simulink model "Main_Project"  (R2016a)
settings: Solver=ode4  StartTime=0.0  StopTime=100  FixedStep=0.001  MaxStep=0.01  RelTol=1e-6
values from neighbouring files (symbols this model uses):
  float =     [waveglider.mat]
  floatABC =     [waveglider.mat]
  gliderABC =     [waveglider.mat]
undefined symbols (not defined in the file or in its folder): magnitude, RAO_Vel
libraries: simulink_extras x8, marine_gnc x4, simulink x4, marine_hydro x1
(part 2 of 3)

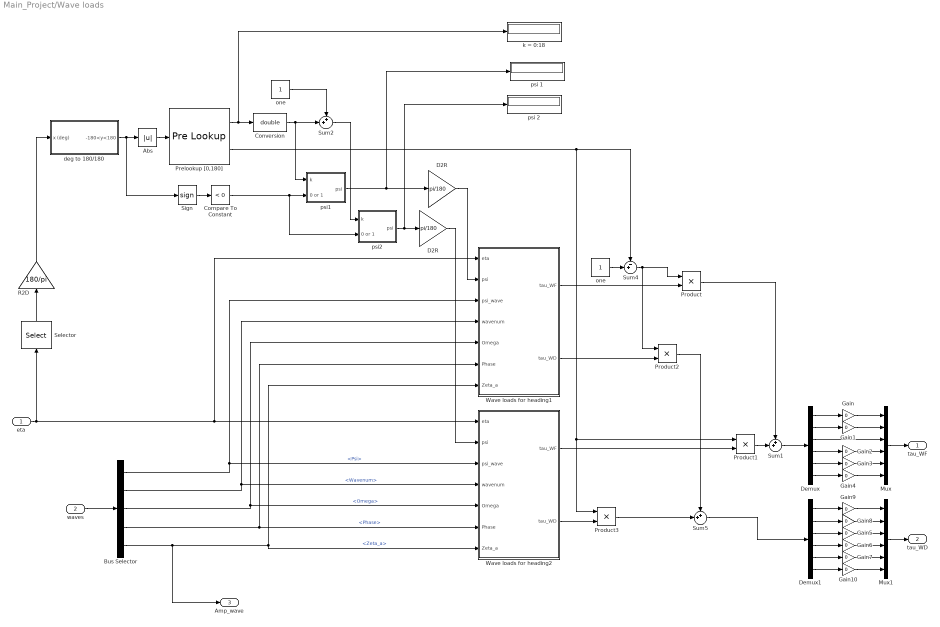
== system Main_Project/Wave loads ==
  eta : Inport
  waves : Inport  Port=2
  Abs : Abs  SaturateOnIntegerOverflow=on
  Bus Selector : BusSelector  OutputSignals=Psi,Wavenum,Omega,Phase,Zeta_a
  Compare To Constant : simulink/Logic and Bit Operations/Compare To Constant  relop=<  const=0  OutDataTypeStr=uint8  ZeroCross=off
  Conversion : DataTypeConversion  OutDataTypeStr=double
  D2R : Gain  Gain=pi/180
  "D2R " : Gain  Gain=pi/180
  Demux : Demux  Outputs=6
  Demux1 : Demux  Outputs=6
  Gain{,1..10} (11 alike) : Gain  Gain=0
  Mux : Mux  Inputs=6
  Mux1 : Mux  Inputs=6
  Prelookup [0,180] : PreLookup  BreakpointsData=[0:10:180]  IndexSearchMethod=Evenly spaced points  BeginIndexSearchUsingPreviousIndexResult=on
  Product{,1..3} (4 alike) : Product  RndMeth=Zero
  R2D : Gain  Gain=180/pi
  Selector : Selector  InputPortWidth=6  IndexOptions=Index vector (dialog)  Indices=[6]  OutputSizes=1
  Sign : Signum
  Sum1 : Sum  Inputs=++|
  Sum2 : Sum  Inputs=++|
  Sum4 : Sum  Inputs=-+|
  Sum5 : Sum  Inputs=++|
  Wave loads for heading1 : Subsystem  mask(Force RAO){ForceRAO_Freq=float.forceRAO.w, WD_Freq=float.driftfrc.w, ForceRAO_Amp=float.forceRAO.amp, ForceRAO_Phase=float.forceRAO.phase, WD_Amp=float.driftfrc.amp, RAO_add_omega_0=on, RAO_add_omega_inf=on}
      mask prompts: ForceRAO_Freq "Vector of frequencies ForceRAO_Freq (rad/s)"; WD_Freq "Vector of frequencies WD_Freq (rad/s)"; ForceRAO_Amp "6DOF Cell array with tables of Amplitudes ForceRAO_Amp"; ForceRAO_Phase "6DOF Cell array with tables of Phases ForceRAO_Phase (rad)"; WD_Amp "6DOF Cell array with tables of Amplitudes WD_Amp"; RAO_add_omega_0 "Add asymptotic RAO values for omega = 0"; RAO_add_omega_inf "Add asymptotic RAO values for omega = inf"
      mask help:
      | Calculate the 6 degrees-of-freedom (DOF) wave-frequency excitation forces tau_WF for a vessel from its Force Response Amplitude Operators (Force RAOs) and a sea state defined by a set of harmonic waves. The block takes the "Waves" bus from the MSS Waves block as input, as well as the vessel low-frequency (LF) motion in terms of the generalized position vector eta and mean surge velocity U. See help for details.
      |
      | Authors: Oyvind N. Smogeli and Thor I. Fossen, 2005-05-03
      mask Help:
      | <b>Part of the Marine Systems Simulator: MSS</b><br>
      | <br>
      | Calculate the 6 degrees-of-freedom (DOF) wave-frequency excitation forces tau_WF
      | for a vessel from its Force Response Amplitude Operators (Force RAOs) and a sea
      | state defined by a set of harmonic waves. The block takes the &quot;Waves&quot; bus from
      | the MSS Waves block as input, as well as the vessel low-frequency (LF) motion in
      | terms of the generalized position vector eta and mean surge velocity U.<p>The Force RAOs are defined in terms of a
      | vector of frequencies (RAO_Freq), a vector of directions (RAO_Dir), a vector of
      | velocities (RAO_Dir), a 6DOF cell array of 3D matrices with amplitudes
      | (RAO_Amp), and a 6DOF cell array of 3D matrices with phases (RAO_Phase), which
      | are all input in the block mask. The first dimension of the 3D matrices
      | corresponds to the frequencies, the second to the directions, and the third to
      | the velocities, such that e.g. the amplitude amp in heave (DOF #3) for frequency
      | number n_f, direction number n_d and velocity number n_v can be found from a =
      | RAO_Amp{3}(n_f, n_d, n_v).</p>
      | <p><b>Inputs:</b></p>
      | <p>Waves:&nbsp;&nbsp;&nbsp;&nbsp;&nbsp;&nbsp;&nbsp;&nbsp;&nbsp;&nbsp;&nbsp; Bus
      | containing the following signals<br>
      | &nbsp;&nbsp;&nbsp; Zeta_a:&nbsp;&nbsp;&nbsp;&nbsp;&nbsp;&nbsp;&nbsp; Vector of harmonic wave amplitudes [m]<br>
      | &nbsp;&nbsp;&nbsp; Omega:&nbsp;&nbsp;&nbsp;&nbsp;&nbsp;&nbsp; Vector of harmonic wave frequencies [rad/s]<br>
      | &nbsp;&nbsp;&nbsp; Phase:&nbsp;&nbsp;&nbsp;&nbsp;&nbsp;&nbsp;&nbsp;&nbsp; Vector of harmonic wave phases (random) [rad]<br>
      | &nbsp;&nbsp;&nbsp; Wavenum:&nbsp;&nbsp;&nbsp; Vector of harmonic wave numbers [1/m]<br>
      | &nbsp;&nbsp;&nbsp; Psi:&nbsp;&nbsp;&nbsp;&nbsp;&nbsp;&nbsp;&nbsp;&nbsp;&nbsp;&nbsp;&nbsp;&nbsp;&nbsp; Vector of harmonic wave directions [rad]</p>
      | <p>eta_LF:&nbsp;&nbsp;&nbsp;&nbsp;&nbsp;&nbsp;&nbsp;&nbsp;&nbsp;&nbsp;&nbsp;
      | Generalized 6DOF n-frame low-frequency position vector [x (m), y (m), z (m),
      | theta (rad), phi (rad), psi (rad)]<br>
      | U:&nbsp;&nbsp;&nbsp;&nbsp;&nbsp;&nbsp;&nbsp;&nbsp;&nbsp;&nbsp;&nbsp;&nbsp;&nbsp;&nbsp;&nbsp;&nbsp;&nbsp;&nbsp;&nbsp;
      | Low-frequency (mean) surge velocity&nbsp; [m/s]</p>
      | <p><b>Outputs:</b></p>
      | <p>tau_WF:&nbsp;&nbsp;&nbsp;&nbsp;&nbsp;&nbsp;&nbsp;&nbsp;&nbsp; Generalized
      | 6DOF h-frame force vector [X (N), Y (N), Z (N), K (Nm), M (Nm), N (Nm)]</p>
      | <p><b>Model validity:</b></p>
      | <p>The validity of the block is dependent on the validity of the given
      | RAO data set.</p>
      | <p>A proper RAO to be used with this block should contain at least 1 velocity, 5
      | directions (e.g. 0, 45, 90, 135 and 180 degrees) and 10-20 frequencies, for all
      | 6 DOF (surge, sway, heave, roll, pitch, yaw).</p>
      | <p>The block performs linear interpolation in frequencies and directions, and
      | uses the data set for the velocity closest to the input velocity (i.e. 'nearest'
      | interpolation in velocity). If the block recieves an input wave frequency or relative
      | wave direction outside the span of the data vectors RAO_Freq or RAO_Dir
      | respectively, the simulation stops and an error is returned. This means that a well-defined
      | RAO must contain data for both 0 and 180 degrees, and for frequencies covering
      | the desired range of wave frequencies. If desired, asymptotic values can be
      | automatically added for zero and infinity frequency to avoid runtime errors if
      | the wave freqeuncy exceeds the values in RAO_Freq (see checkboxes in the mask). </p>
      | <p>IMPORTANT NOTE: The RAO theory upon which this block is based is in reality
      | only valid when the vessel low-frequency (h-frame) motion is a constant surge
      | velocity only, and the vessel is performing wave-frequency oscillations about
      | the steadily translating h-frame.This means that the outputs from the block when
      | manoeuvering -- i.e. changing the surge velocity and/or yaw angle -- must be
      | interpreted with some care. A jump in the output must be expected when changing
      | between two velocity data sets, and frequency warping expected when changing the
      | yaw angle (due to interpolation in the phase). It is therefore recommended to
      | use backlash on the input velocity to avoid transient switching, and a quantized
      | yaw angle with backlash. The latter will lead to jump in the ouput when the yaw
      | angle changes from one quantized value to another, but will give better results
      | when keeping within one quantizer interval. The quantized yaw angle with
      | backlash and velocity with backlash are available as options via checkboxes in
      | the mask. If either of these are activated, proper values for the yaw
      | quantization interval, yaw backlash width, and the the speed backlash width
      | respectively must be set. Typical values could be a yaw quantization interval of
      | 5 degrees, yaw backlash width of 1/4-1/5 of the quantization interval, and speed
      | backlash width of 1 m/s. To avoid the most rapid transients when switching
      | between data sets, output smoothing is available as an option in the mask. If
      | this is enabled, the output during a transent is rate limited according to the
      | fastest recorded signal rate during normal operation.</p>
      | <p><b>Example mask input:</b></p><p>
      | As an example, the format of the mask input for 2 velocities, 3 directions and 5
      | frequencies is as follows:<p>RAO_Freq = [f1 f2 f3 f4 f5]<br>
      | RAO_Dir = [d1 d2 d3]<br>
      | RAO_Vel = [v1 v2]<p>Surge:<br>
      | RAO_Amp{1}(:,:,1)&nbsp; = [a1_111 a1_121 a1_131; a1_211 a1_221 a1_231; a1_311
      | a1_321 a1_331; a1_411 a1_421 a1_431; a1_511 a1_521 a1_531]<br>
      | RAO_Amp{1}(:,:,2)&nbsp; = [a1_112 a1_122 a1_132; a1_212 a1_222 a1_232; a1_312
      | a1_322 a1_332; a1_412 a1_422 a1_432; a1_512 a1_522 a1_532]<br>
      | RAO_Phase{1}(:,:,1) = [p1_111 p1_121 p1_131; p1_211 p1_221 p1_231; p1_311 p1_321
      | p1_331; p1_411 p1_421 p1_431; p1_511 p1_521 p1_531]<br>
      | RAO_Phase{1}(:,:,2) = [p1_112 p1_122 p1_132; p1_212 p1_222 p1_232; p1_312 p1_322
      | p1_332; p1_412 p1_422 p1_432; p1_512 p1_522 p1_532]<p>Sway:<br>
      | RAO_Amp{2}(:,:,1)&nbsp; = [a2_111 a2_121 a2_131; a2_211 a2_221 a2_231; a2_311
      | a2_321 a2_331; a2_411 a2_421 a2_431; a2_511 a2_521 a2_531]<br>
      | RAO_Amp{2}(:,:,2)&nbsp; = [a2_112 a2_122 a2_132; a2_212 a2_222 a2_232; a2_312
      | a2_322 a2_332; a2_412 a2_422 a2_432; a2_512 a2_522 a2_532]<br>
      | RAO_Phase{2}(:,:,1) = [p2_111 p2_121 p2_131; p2_211 p2_221 p2_231; p2_311 p2_321
      | p2_331; p2_411 p2_421 p2_431; p2_511 p2_521 p2_531]<br>
      | RAO_Phase{2}(:,:,2) = [p2_112 p2_122 p2_132; p2_212 p2_222 p2_232; p2_312 p2_322
      | p2_332; p2_412 p2_422 p2_432; p2_512 p2_522 p2_532]<p>...<p>Yaw:<br>
      | RAO_Amp{6}(:,:,1)&nbsp; = [a6_111 a6_121 a6_131; a6_211 a6_221 a6_231; a6_311
      | a6_321 a6_331; a6_411 a6_421 a6_431; a6_511 a6_521 a6_531]<br>
      | RAO_Amp{6}(:,:,2)&nbsp; = [a6_112 a6_122 a6_132; a6_212 a6_222 a6_232; a6_312
      | a6_322 a6_332; a6_412 a6_422 a6_432; a6_512 a6_522 a6_532]<br>
      | RAO_Phase{6}(:,:,1) = [p6_111 p6_121 p6_131; p6_211 p6_221 p6_231; p6_311 p6_321
      | p6_331; p6_411 p6_421 p6_431; p6_511 p6_521 p6_531]<br>
      | RAO_Phase{6}(:,:,2) = [p6_112 p6_122 p6_132; p6_212 p6_222 p6_232; p6_312 p6_322
      | p6_332; p6_412 p6_422 p6_432; p6_512 p6_522 p6_532]<p>where now for example the
      | amplitude and phase in sway (DOF 2) for frequency f5, direction d3 and velocity
      | v1 are given by RAO_Amp{2}(5,3,1) = a2_531 and RAO_Phase{2}(5,3,1) = p2_531.<p>
      | <b>Copyright (C) NTNU 2005</b></p>
      | <p><b>Author:</b> Oyvind N. Smogeli, 2005-05-03</p>
  Wave loads for heading2 : Subsystem  mask(Force RAO){ForceRAO_Freq=float.forceRAO.w, RAO_Vel=float.velocities, ForceRAO_Amp=float.forceRAO.amp, ForceRAO_Phase=float.forceRAO.phase, WD_Amp=float.driftfrc.amp, RAO_add_omega_0=on, RAO_add_omega_inf=on}
      mask prompts: ForceRAO_Freq "Vector of frequencies ForceRAO_Freq (rad/s)"; RAO_Vel "Vector of velocities RAO_Vel (m/s)"; ForceRAO_Amp "6DOF Cell array with tables of Amplitudes ForceRAO_Amp"; ForceRAO_Phase "6DOF Cell array with tables of Phases ForceRAO_Phase (rad)"; WD_Amp "6DOF Cell array with tables of Amplitudes WD_Amp"; RAO_add_omega_0 "Add asymptotic RAO values for omega = 0"; RAO_add_omega_inf "Add asymptotic RAO values for omega = inf"
      mask help:
      | Calculate the 6 degrees-of-freedom (DOF) wave-frequency excitation forces tau_WF for a vessel from its Force Response Amplitude Operators (Force RAOs) and a sea state defined by a set of harmonic waves. The block takes the "Waves" bus from the MSS Waves block as input, as well as the vessel low-frequency (LF) motion in terms of the generalized position vector eta and mean surge velocity U. See help for details.
      |
      | Authors: Oyvind N. Smogeli and Thor I. Fossen, 2005-05-03
      mask Help:
      | <b>Part of the Marine Systems Simulator: MSS</b><br>
      | <br>
      | Calculate the 6 degrees-of-freedom (DOF) wave-frequency excitation forces tau_WF
      | for a vessel from its Force Response Amplitude Operators (Force RAOs) and a sea
      | state defined by a set of harmonic waves. The block takes the &quot;Waves&quot; bus from
      | the MSS Waves block as input, as well as the vessel low-frequency (LF) motion in
      | terms of the generalized position vector eta and mean surge velocity U.<p>The Force RAOs are defined in terms of a
      | vector of frequencies (RAO_Freq), a vector of directions (RAO_Dir), a vector of
      | velocities (RAO_Dir), a 6DOF cell array of 3D matrices with amplitudes
      | (RAO_Amp), and a 6DOF cell array of 3D matrices with phases (RAO_Phase), which
      | are all input in the block mask. The first dimension of the 3D matrices
      | corresponds to the frequencies, the second to the directions, and the third to
      | the velocities, such that e.g. the amplitude amp in heave (DOF #3) for frequency
      | number n_f, direction number n_d and velocity number n_v can be found from a =
      | RAO_Amp{3}(n_f, n_d, n_v).</p>
      | <p><b>Inputs:</b></p>
      | <p>Waves:&nbsp;&nbsp;&nbsp;&nbsp;&nbsp;&nbsp;&nbsp;&nbsp;&nbsp;&nbsp;&nbsp; Bus
      | containing the following signals<br>
      | &nbsp;&nbsp;&nbsp; Zeta_a:&nbsp;&nbsp;&nbsp;&nbsp;&nbsp;&nbsp;&nbsp; Vector of harmonic wave amplitudes [m]<br>
      | &nbsp;&nbsp;&nbsp; Omega:&nbsp;&nbsp;&nbsp;&nbsp;&nbsp;&nbsp; Vector of harmonic wave frequencies [rad/s]<br>
      | &nbsp;&nbsp;&nbsp; Phase:&nbsp;&nbsp;&nbsp;&nbsp;&nbsp;&nbsp;&nbsp;&nbsp; Vector of harmonic wave phases (random) [rad]<br>
      | &nbsp;&nbsp;&nbsp; Wavenum:&nbsp;&nbsp;&nbsp; Vector of harmonic wave numbers [1/m]<br>
      | &nbsp;&nbsp;&nbsp; Psi:&nbsp;&nbsp;&nbsp;&nbsp;&nbsp;&nbsp;&nbsp;&nbsp;&nbsp;&nbsp;&nbsp;&nbsp;&nbsp; Vector of harmonic wave directions [rad]</p>
      | <p>eta_LF:&nbsp;&nbsp;&nbsp;&nbsp;&nbsp;&nbsp;&nbsp;&nbsp;&nbsp;&nbsp;&nbsp;
      | Generalized 6DOF n-frame low-frequency position vector [x (m), y (m), z (m),
      | theta (rad), phi (rad), psi (rad)]<br>
      | U:&nbsp;&nbsp;&nbsp;&nbsp;&nbsp;&nbsp;&nbsp;&nbsp;&nbsp;&nbsp;&nbsp;&nbsp;&nbsp;&nbsp;&nbsp;&nbsp;&nbsp;&nbsp;&nbsp;
      | Low-frequency (mean) surge velocity&nbsp; [m/s]</p>
      | <p><b>Outputs:</b></p>
      | <p>tau_WF:&nbsp;&nbsp;&nbsp;&nbsp;&nbsp;&nbsp;&nbsp;&nbsp;&nbsp; Generalized
      | 6DOF h-frame force vector [X (N), Y (N), Z (N), K (Nm), M (Nm), N (Nm)]</p>
      | <p><b>Model validity:</b></p>
      | <p>The validity of the block is dependent on the validity of the given
      | RAO data set.</p>
      | <p>A proper RAO to be used with this block should contain at least 1 velocity, 5
      | directions (e.g. 0, 45, 90, 135 and 180 degrees) and 10-20 frequencies, for all
      | 6 DOF (surge, sway, heave, roll, pitch, yaw).</p>
      | <p>The block performs linear interpolation in frequencies and directions, and
      | uses the data set for the velocity closest to the input velocity (i.e. 'nearest'
      | interpolation in velocity). If the block recieves an input wave frequency or relative
      | wave direction outside the span of the data vectors RAO_Freq or RAO_Dir
      | respectively, the simulation stops and an error is returned. This means that a well-defined
      | RAO must contain data for both 0 and 180 degrees, and for frequencies covering
      | the desired range of wave frequencies. If desired, asymptotic values can be
      | automatically added for zero and infinity frequency to avoid runtime errors if
      | the wave freqeuncy exceeds the values in RAO_Freq (see checkboxes in the mask). </p>
      | <p>IMPORTANT NOTE: The RAO theory upon which this block is based is in reality
      | only valid when the vessel low-frequency (h-frame) motion is a constant surge
      | velocity only, and the vessel is performing wave-frequency oscillations about
      | the steadily translating h-frame.This means that the outputs from the block when
      | manoeuvering -- i.e. changing the surge velocity and/or yaw angle -- must be
      | interpreted with some care. A jump in the output must be expected when changing
      | between two velocity data sets, and frequency warping expected when changing the
      | yaw angle (due to interpolation in the phase). It is therefore recommended to
      | use backlash on the input velocity to avoid transient switching, and a quantized
      | yaw angle with backlash. The latter will lead to jump in the ouput when the yaw
      | angle changes from one quantized value to another, but will give better results
      | when keeping within one quantizer interval. The quantized yaw angle with
      | backlash and velocity with backlash are available as options via checkboxes in
      | the mask. If either of these are activated, proper values for the yaw
      | quantization interval, yaw backlash width, and the the speed backlash width
      | respectively must be set. Typical values could be a yaw quantization interval of
      | 5 degrees, yaw backlash width of 1/4-1/5 of the quantization interval, and speed
      | backlash width of 1 m/s. To avoid the most rapid transients when switching
      | between data sets, output smoothing is available as an option in the mask. If
      | this is enabled, the output during a transent is rate limited according to the
      | fastest recorded signal rate during normal operation.</p>
      | <p><b>Example mask input:</b></p><p>
      | As an example, the format of the mask input for 2 velocities, 3 directions and 5
      | frequencies is as follows:<p>RAO_Freq = [f1 f2 f3 f4 f5]<br>
      | RAO_Dir = [d1 d2 d3]<br>
      | RAO_Vel = [v1 v2]<p>Surge:<br>
      | RAO_Amp{1}(:,:,1)&nbsp; = [a1_111 a1_121 a1_131; a1_211 a1_221 a1_231; a1_311
      | a1_321 a1_331; a1_411 a1_421 a1_431; a1_511 a1_521 a1_531]<br>
      | RAO_Amp{1}(:,:,2)&nbsp; = [a1_112 a1_122 a1_132; a1_212 a1_222 a1_232; a1_312
      | a1_322 a1_332; a1_412 a1_422 a1_432; a1_512 a1_522 a1_532]<br>
      | RAO_Phase{1}(:,:,1) = [p1_111 p1_121 p1_131; p1_211 p1_221 p1_231; p1_311 p1_321
      | p1_331; p1_411 p1_421 p1_431; p1_511 p1_521 p1_531]<br>
      | RAO_Phase{1}(:,:,2) = [p1_112 p1_122 p1_132; p1_212 p1_222 p1_232; p1_312 p1_322
      | p1_332; p1_412 p1_422 p1_432; p1_512 p1_522 p1_532]<p>Sway:<br>
      | RAO_Amp{2}(:,:,1)&nbsp; = [a2_111 a2_121 a2_131; a2_211 a2_221 a2_231; a2_311
      | a2_321 a2_331; a2_411 a2_421 a2_431; a2_511 a2_521 a2_531]<br>
      | RAO_Amp{2}(:,:,2)&nbsp; = [a2_112 a2_122 a2_132; a2_212 a2_222 a2_232; a2_312
      | a2_322 a2_332; a2_412 a2_422 a2_432; a2_512 a2_522 a2_532]<br>
      | RAO_Phase{2}(:,:,1) = [p2_111 p2_121 p2_131; p2_211 p2_221 p2_231; p2_311 p2_321
      | p2_331; p2_411 p2_421 p2_431; p2_511 p2_521 p2_531]<br>
      | RAO_Phase{2}(:,:,2) = [p2_112 p2_122 p2_132; p2_212 p2_222 p2_232; p2_312 p2_322
      | p2_332; p2_412 p2_422 p2_432; p2_512 p2_522 p2_532]<p>...<p>Yaw:<br>
      | RAO_Amp{6}(:,:,1)&nbsp; = [a6_111 a6_121 a6_131; a6_211 a6_221 a6_231; a6_311
      | a6_321 a6_331; a6_411 a6_421 a6_431; a6_511 a6_521 a6_531]<br>
      | RAO_Amp{6}(:,:,2)&nbsp; = [a6_112 a6_122 a6_132; a6_212 a6_222 a6_232; a6_312
      | a6_322 a6_332; a6_412 a6_422 a6_432; a6_512 a6_522 a6_532]<br>
      | RAO_Phase{6}(:,:,1) = [p6_111 p6_121 p6_131; p6_211 p6_221 p6_231; p6_311 p6_321
      | p6_331; p6_411 p6_421 p6_431; p6_511 p6_521 p6_531]<br>
      | RAO_Phase{6}(:,:,2) = [p6_112 p6_122 p6_132; p6_212 p6_222 p6_232; p6_312 p6_322
      | p6_332; p6_412 p6_422 p6_432; p6_512 p6_522 p6_532]<p>where now for example the
      | amplitude and phase in sway (DOF 2) for frequency f5, direction d3 and velocity
      | v1 are given by RAO_Amp{2}(5,3,1) = a2_531 and RAO_Phase{2}(5,3,1) = p2_531.<p>
      | <b>Copyright (C) NTNU 2005</b></p>
      | <p><b>Author:</b> Oyvind N. Smogeli, 2005-05-03</p>
  deg to 180/180 : Subsystem  AncestorBlock=marine_gnc/Utilities/Math Operations/deg to 180//180  mask(deg to 180/180){}
      mask help: Converts an angle in deg to +- 180 deg
      mask Display: disp('[0 360] to [-180 180]')
  k = 0:18 : Display
  one : Constant
  "one " : Constant
  psi 1 : Display
  psi 2 : Display
  psi1 : Subsystem
  psi2 : Subsystem
  tau_WF : Outport
  tau_WD : Outport  Port=2
  Amp_wave : Outport  Port=3
  wires:
  R2D/1 -> deg to 180/180/1(x (deg))
  Selector/1 -> R2D/1
  waves/1 -> Bus Selector/1
  "D2R "/1 -> Wave loads for heading2/2(psi)
  D2R/1 -> Wave loads for heading1/2(psi)
  psi2/1(psi) -> psi 2/1, "D2R "/1
  Conversion/1 -> psi1/1(k), Sum2/2
  Prelookup [0,180]/2 -> Sum4/1, Product1/1, Product3/1
  psi1/1(psi) -> psi 1/1, D2R/1
  Compare To Constant/1 -> psi2/2(0 or 1), psi1/2(0 or 1)
  Sign/1 -> Compare To Constant/1
  Abs/1 -> Prelookup [0,180]/1
  deg to 180/180/1(-180<y<180) -> Sign/1, Abs/1
  Sum2/1 -> psi2/1(k)
  one/1 -> Sum2/1
  Prelookup [0,180]/1 -> k = 0:18/1, Conversion/1
  Product2/1 -> Sum5/1
  Product3/1 -> Sum5/2
  Wave loads for heading1/2(tau_WD) -> Product2/2
  Sum4/1 -> Product2/1, Product/1
  "one "/1 -> Sum4/2
  Product1/1 -> Sum1/2
  Product/1 -> Sum1/1
  Wave loads for heading1/1(tau_WF) -> Product/2
  Bus Selector/5 -> Amp_wave/1, Wave loads for heading2/7(Zeta_a), Wave loads for heading1/7(Zeta_a)  "<Zeta_a>"
  Bus Selector/4 -> Wave loads for heading2/6(Phase), Wave loads for heading1/6(Phase)  "<Phase>"
  Bus Selector/3 -> Wave loads for heading2/5(Omega), Wave loads for heading1/5(Omega)  "<Omega>"
  Bus Selector/2 -> Wave loads for heading2/4(wavenum), Wave loads for heading1/4(wavenum)  "<Wavenum>"
  Bus Selector/1 -> Wave loads for heading2/3(psi_wave), Wave loads for heading1/3(psi_wave)  "<Psi>"
  eta/1 -> Selector/1, Wave loads for heading2/1(eta), Wave loads for heading1/1(eta)
  Wave loads for heading2/2(tau_WD) -> Product3/2
  Wave loads for heading2/1(tau_WF) -> Product1/2
  Sum1/1 -> Demux/1
  Mux/1 -> tau_WF/1
  Demux/3 -> Mux/3
  Demux/1 -> Gain/1
  Demux/2 -> Gain1/1
  Demux/4 -> Gain2/1
  Demux/5 -> Gain3/1
  Demux/6 -> Gain4/1
  Sum5/1 -> Demux1/1
  Mux1/1 -> tau_WD/1
  Demux1/3 -> Gain5/1
  Demux1/1 -> Gain9/1
  Demux1/2 -> Gain8/1
  Demux1/4 -> Gain6/1
  Demux1/5 -> Gain7/1
  Demux1/6 -> Gain10/1
  Gain/1 -> Mux/1
  Gain1/1 -> Mux/2
  Gain2/1 -> Mux/4
  Gain3/1 -> Mux/5
  Gain4/1 -> Mux/6
  Gain5/1 -> Mux1/3
  Gain6/1 -> Mux1/4
  Gain7/1 -> Mux1/5
  Gain8/1 -> Mux1/2
  Gain9/1 -> Mux1/1
  Gain10/1 -> Mux1/6

== system Main_Project/Waves ==
  Bus Creator : BusCreator  Inputs=5
  Omega : Constant  Value=Omega
  Phase : Constant  Value=Phase
  Psi : Constant  Value=Psi
  Wavenum : Constant  Value=Wavenum
  Zeta_a : Constant  Value=Zeta_a
  "wave direction " : Constant  Value=psi_mean
  Waves : Outport
  wave direction : Outport  Port=2
  wires:
  "wave direction "/1 -> wave direction/1
  Wavenum/1 -> Bus Creator/4  "Wavenum"
  Zeta_a/1 -> Bus Creator/3  "Zeta_a"
  Bus Creator/1 -> Waves/1
  Omega/1 -> Bus Creator/1  "Omega"
  Psi/1 -> Bus Creator/2  "Psi"
  Phase/1 -> Bus Creator/5  "Phase"

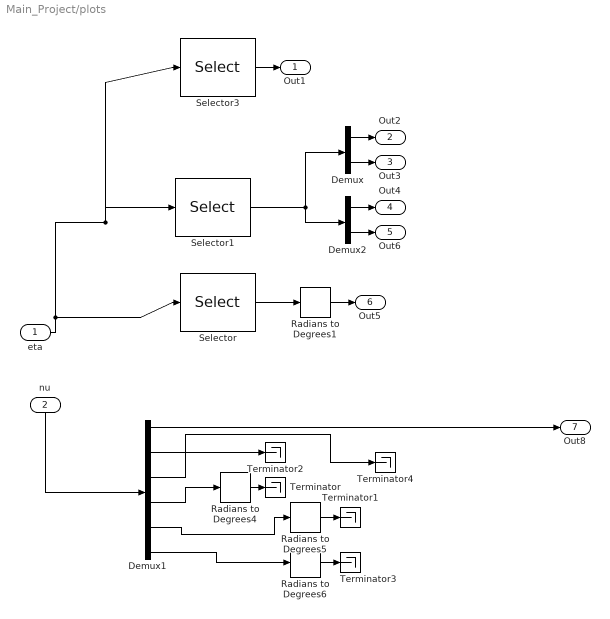
== system Main_Project/plots ==
  eta : Inport
  nu : Inport  Port=2
  Demux : Demux  Outputs=2
  Demux1 : Demux  Outputs=6
  Demux2 : Demux  Outputs=2
  Radians to Degrees{1,4..6} (4 alike) : simulink_extras/Transformations/Radians to Degrees
  Selector : Selector  InputPortWidth=6  IndexOptions=Index vector (dialog)  Indices=[6 ]  OutputSizes=1
  Selector1 : Selector  InputPortWidth=6  IndexOptions=Index vector (dialog)  Indices=[1 2]  OutputSizes=1
  Selector3 : Selector  InputPortWidth=6  IndexOptions=Index vector (dialog)  Indices=[3]  OutputSizes=1
  Terminator{,1..4} (5 alike) : Terminator
  Out1 : Outport
  Out2 : Outport  Port=2
  Out3 : Outport  Port=3
  Out4 : Outport  Port=4
  Out6 : Outport  Port=5
  Out5 : Outport  Port=6
  Out8 : Outport  Port=7
  wires:
  eta/1 -> Selector3/1, Selector1/1, Selector/1
  Selector/1 -> Radians to Degrees1/1
  Selector1/1 -> Demux/1, Demux2/1
  Selector3/1 -> Out1/1
  Demux/1 -> Out2/1
  Demux/2 -> Out3/1
  Radians to Degrees1/1 -> Out5/1
  nu/1 -> Demux1/1
  Demux1/4 -> Radians to Degrees4/1
  Demux1/5 -> Radians to Degrees5/1
  Demux1/6 -> Radians to Degrees6/1
  Demux1/1 -> Out8/1
  Radians to Degrees4/1 -> Terminator/1
  Radians to Degrees5/1 -> Terminator1/1
  Demux2/1 -> Out4/1
  Demux2/2 -> Out6/1
  Demux1/2 -> Terminator2/1
  Radians to Degrees6/1 -> Terminator3/1
  Demux1/3 -> Terminator4/1

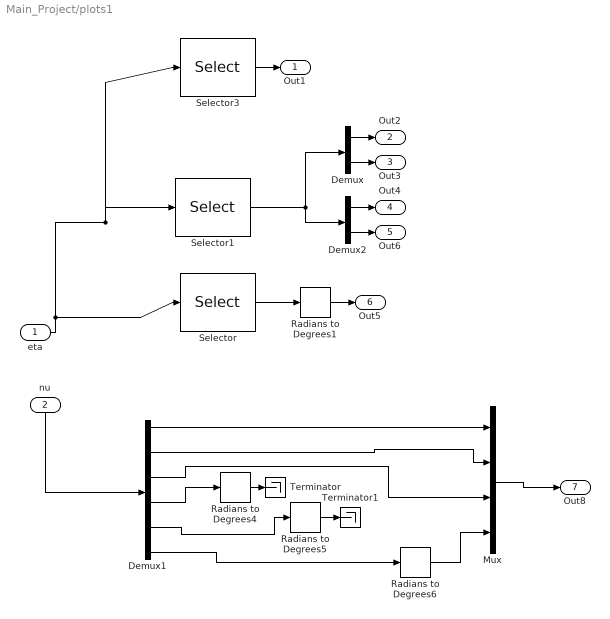
== system Main_Project/plots1 ==
  eta : Inport
  nu : Inport  Port=2
  Demux : Demux  Outputs=2
  Demux1 : Demux  Outputs=6
  Demux2 : Demux  Outputs=2
  Mux : Mux
  Radians to Degrees{1,4..6} (4 alike) : simulink_extras/Transformations/Radians to Degrees
  Selector : Selector  InputPortWidth=6  IndexOptions=Index vector (dialog)  Indices=[6 ]  OutputSizes=1
  Selector1 : Selector  InputPortWidth=6  IndexOptions=Index vector (dialog)  Indices=[1 2]  OutputSizes=1
  Selector3 : Selector  InputPortWidth=6  IndexOptions=Index vector (dialog)  Indices=[3]  OutputSizes=1
  Terminator : Terminator
  Terminator1 : Terminator
  Out1 : Outport
  Out2 : Outport  Port=2
  Out3 : Outport  Port=3
  Out4 : Outport  Port=4
  Out6 : Outport  Port=5
  Out5 : Outport  Port=6
  Out8 : Outport  Port=7
  wires:
  eta/1 -> Selector3/1, Selector1/1, Selector/1
  Selector/1 -> Radians to Degrees1/1
  Selector1/1 -> Demux/1, Demux2/1
  Selector3/1 -> Out1/1
  Demux/1 -> Out2/1
  Demux/2 -> Out3/1
  Radians to Degrees1/1 -> Out5/1
  nu/1 -> Demux1/1
  Demux1/1 -> Mux/1
  Demux1/2 -> Mux/2
  Demux1/3 -> Mux/3
  Demux1/4 -> Radians to Degrees4/1
  Demux1/5 -> Radians to Degrees5/1
  Demux1/6 -> Radians to Degrees6/1
  Radians to Degrees6/1 -> Mux/4
  Mux/1 -> Out8/1
  Radians to Degrees4/1 -> Terminator/1
  Radians to Degrees5/1 -> Terminator1/1
  Demux2/1 -> Out4/1
  Demux2/2 -> Out6/1

== system Main_Project/quardratic damping ==
  nu_r : Inport
  Abs : Abs
  Demux : Demux  Outputs=6
  Gain{,1..4} (5 alike) : Gain  Gain=0
  Gain5 : Gain  Gain=0.5*0.7*1024*0.2868
  Mux : Mux  Inputs=6
  Product : Product
  d(vr) : Outport
  wires:
  Mux/1 -> d(vr)/1
  nu_r/1 -> Demux/1
  Gain5/1 -> Mux/2
  Gain/1 -> Mux/1
  Demux/1 -> Gain/1
  Gain1/1 -> Mux/3
  Demux/3 -> Gain1/1
  Gain2/1 -> Mux/4
  Demux/4 -> Gain2/1
  Gain3/1 -> Mux/5
  Demux/5 -> Gain3/1
  Gain4/1 -> Mux/6
  Demux/6 -> Gain4/1
  Abs/1 -> Product/1
  Demux/2 -> Abs/1, Product/2
  Product/1 -> Gain5/1

== system Main_Project/rad2deg ==
  In : Inport
  Gain : Gain  Gain=k  SaturateOnIntegerOverflow=on  OutDataTypeStr=Inherit: Same as input  ParamDataTypeStr=Inherit: Same as input
  Out : Outport
  wires:
  Gain/1 -> Out/1
  In/1 -> Gain/1

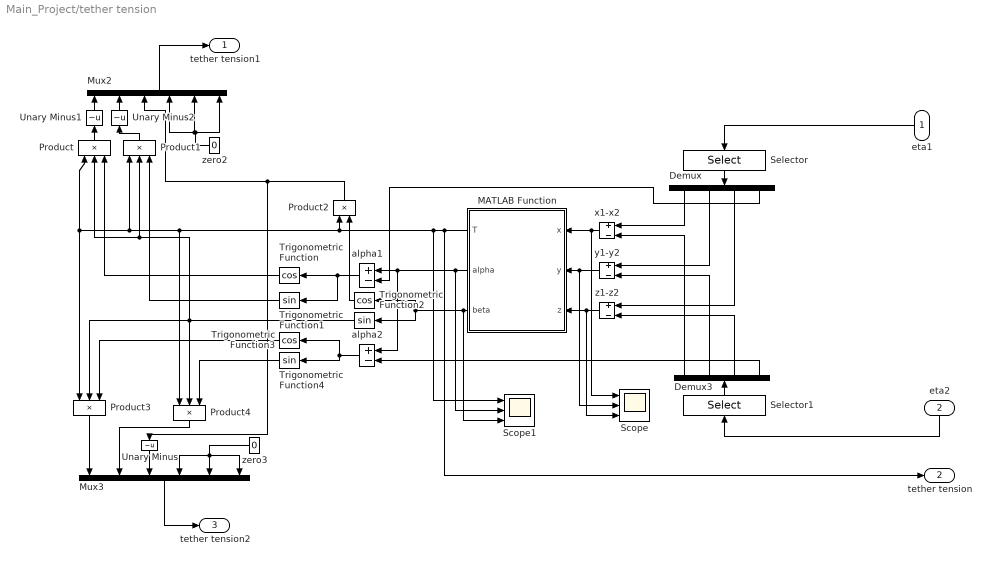
== system Main_Project/tether tension ==
  eta1 : Inport
  eta2 : Inport  Port=2
  "                " : Trigonometry
  Demux : Demux
  Demux3 : Demux
  MATLAB Function : MATLAB Function  TreatAsAtomicUnit=on
  Mux2 : Mux  Inputs=6
  Mux3 : Mux  Inputs=6
  Product{,1,3..4} (4 alike) : Product  Inputs=3
  Product2 : Product
  Scope : Scope  NumInputPorts=3
  Scope1 : Scope  NumInputPorts=3
  Selector : Selector  InputPortWidth=6  IndexOptions=Index vector (dialog)  Indices=[1 2 3 6]  OutputSizes=1
  Selector1 : Selector  InputPortWidth=6  IndexOptions=Index vector (dialog)  Indices=[1 2 3 6]  OutputSizes=1
  Trigonometric Function : Trigonometry  Operator=cos
  Trigonometric Function1 : Trigonometry
  Trigonometric Function2 : Trigonometry  Operator=cos
  Trigonometric Function3 : Trigonometry  Operator=cos
  Trigonometric Function4 : Trigonometry
  Unary Minus : UnaryMinus
  Unary Minus1 : UnaryMinus
  Unary Minus2 : UnaryMinus
  alpha1 : Sum  Inputs=+-
  alpha2 : Sum  Inputs=+-
  x1-x2 : Sum  Inputs=+-
  y1-y2 : Sum  Inputs=+-
  z1-z2 : Sum  Inputs=+-
  zero2 : Constant  Value=0
  zero3 : Constant  Value=0
  tether tension1 : Outport
  tether tension : Outport  Port=2
  tether tension2 : Outport  Port=3
  wires:
  Product1/1 -> Unary Minus2/1
  Unary Minus2/1 -> Mux2/2
  Product/1 -> Unary Minus1/1
  Unary Minus1/1 -> Mux2/1
  y1-y2/1 -> Scope/2, MATLAB Function/2(y)
  x1-x2/1 -> Scope/1, MATLAB Function/1(x)
  z1-z2/1 -> Scope/3, MATLAB Function/3(z)
  Demux3/4 -> alpha2/2
  zero2/1 -> Mux2/4, Mux2/5, Mux2/6
  Product4/1 -> Mux3/2
  zero3/1 -> Mux3/6, Mux3/5, Mux3/4
  Trigonometric Function3/1 -> Product3/3
  Mux3/1 -> tether tension2/1
  MATLAB Function/1(T) -> Scope1/1, Product2/1, Product4/1, Product1/1, Product/1, Product3/1, tether tension/1
  alpha1/1 -> Trigonometric Function/1, Trigonometric Function1/1
  "                "/1 -> Product1/2, Product/2, Product3/2, Product4/2
  Product3/1 -> Mux3/1
  Trigonometric Function/1 -> Product/3
  Trigonometric Function1/1 -> Product1/3
  eta1/1 -> Selector/1
  alpha2/1 -> Trigonometric Function4/1, Trigonometric Function3/1
  eta2/1 -> Selector1/1
  Demux3/3 -> z1-z2/2
  Demux/3 -> z1-z2/1
  Demux3/2 -> y1-y2/2
  Demux/2 -> y1-y2/1
  Demux3/1 -> x1-x2/2
  Demux/1 -> x1-x2/1
  Unary Minus/1 -> Mux3/3
  Mux2/1 -> tether tension1/1
  MATLAB Function/2(alpha) -> Scope1/2, alpha1/1, alpha2/1
  Demux/4 -> alpha1/2
  MATLAB Function/3(beta) -> Scope1/3, "                "/1, Trigonometric Function2/1
  Trigonometric Function2/1 -> Product2/2
  Trigonometric Function4/1 -> Product4/3
  Product2/1 -> Unary Minus/1, Mux2/3
  Selector/1 -> Demux/1
  Selector1/1 -> Demux3/1

== system Main_Project/6 DOF transformation/Euler angles to rotation matrix1 ==
  theta : Inport
  Mux : Mux  Inputs=2
  Mux2 : Mux  Inputs=9
  R11 : Fcn  Expr=u(6)*u(5)
  R12 : Fcn  Expr=u(6)*u(2)*u(1)-u(3)*u(4)
  R13 : Fcn  Expr=u(4)*u(2)*u(6)+u(3)*u(1)
  "R21 " : Fcn  Expr=u(3)*u(5)
  R22 : Fcn  Expr=u(3)*u(2)*u(1)+u(6)*u(4)
  R23 : Fcn  Expr=u(3)*u(2)*u(4)-u(6)*u(1)
  "R31 " : Fcn  Expr=-u(2)
  R32 : Fcn  Expr=u(5)*u(1)
  R33 : Fcn  Expr=u(5)*u(4)
  Reshape 9x1->3x3 : Reshape  OutputDimensionality=Customize  OutputDimensions=[3,3]
  cos(theta) : Trigonometry  Operator=cos
  sin(theta) : Trigonometry
  Rzyx : Outport  InitialOutput=0
  wires:
  R33/1 -> Mux2/9
  R32/1 -> Mux2/6
  "R21 "/1 -> Mux2/2
  "R31 "/1 -> Mux2/3
  R12/1 -> Mux2/4
  R22/1 -> Mux2/5
  R13/1 -> Mux2/7
  R23/1 -> Mux2/8
  Mux/1 -> R12/1, "R21 "/1, R11/1, "R31 "/1, R22/1, R23/1, R33/1, R13/1, R32/1
  theta/1 -> cos(theta)/1, sin(theta)/1
  cos(theta)/1 -> Mux/2
  sin(theta)/1 -> Mux/1
  Reshape 9x1->3x3/1 -> Rzyx/1
  Mux2/1 -> Reshape 9x1->3x3/1
  R11/1 -> Mux2/1

== system Main_Project/6 DOF transformation1/Euler angles to rotation matrix1 ==
  theta : Inport
  Mux : Mux  Inputs=2
  Mux2 : Mux  Inputs=9
  R11 : Fcn  Expr=u(6)*u(5)
  R12 : Fcn  Expr=u(6)*u(2)*u(1)-u(3)*u(4)
  R13 : Fcn  Expr=u(4)*u(2)*u(6)+u(3)*u(1)
  "R21 " : Fcn  Expr=u(3)*u(5)
  R22 : Fcn  Expr=u(3)*u(2)*u(1)+u(6)*u(4)
  R23 : Fcn  Expr=u(3)*u(2)*u(4)-u(6)*u(1)
  "R31 " : Fcn  Expr=-u(2)
  R32 : Fcn  Expr=u(5)*u(1)
  R33 : Fcn  Expr=u(5)*u(4)
  Reshape 9x1->3x3 : Reshape  OutputDimensionality=Customize  OutputDimensions=[3,3]
  cos(theta) : Trigonometry  Operator=cos
  sin(theta) : Trigonometry
  Rzyx : Outport  InitialOutput=0
  wires:
  R33/1 -> Mux2/9
  R32/1 -> Mux2/6
  "R21 "/1 -> Mux2/2
  "R31 "/1 -> Mux2/3
  R12/1 -> Mux2/4
  R22/1 -> Mux2/5
  R13/1 -> Mux2/7
  R23/1 -> Mux2/8
  Mux/1 -> R12/1, "R21 "/1, R11/1, "R31 "/1, R22/1, R23/1, R33/1, R13/1, R32/1
  theta/1 -> cos(theta)/1, sin(theta)/1
  cos(theta)/1 -> Mux/2
  sin(theta)/1 -> Mux/1
  Reshape 9x1->3x3/1 -> Rzyx/1
  Mux2/1 -> Reshape 9x1->3x3/1
  R11/1 -> Mux2/1

== system Main_Project/Current speed trans/current1 ==
  beta_c(rad) : Inport
  V_c(m/s) : Inport  Port=2
  Mux : Mux  Inputs=6
  Product : Product  RndMeth=Zero
  Product1 : Product  RndMeth=Zero
  cos : Trigonometry  Operator=cos
  sin : Trigonometry
  zero : Constant  Value=0
  nu_c : Outport
  wires:
  Mux/1 -> nu_c/1
  zero/1 -> Mux/6, Mux/5, Mux/4, Mux/3
  Product1/1 -> Mux/2
  Product/1 -> Mux/1
  V_c(m/s)/1 -> Product/2, Product1/2
  cos/1 -> Product/1
  sin/1 -> Product1/1
  beta_c(rad)/1 -> cos/1, sin/1

== system Main_Project/Current speed trans1/current1 ==
  beta_c(rad) : Inport
  V_c(m/s) : Inport  Port=2
  Mux : Mux  Inputs=6
  Product : Product  RndMeth=Zero
  Product1 : Product  RndMeth=Zero
  cos : Trigonometry  Operator=cos
  sin : Trigonometry
  zero : Constant  Value=0
  nu_c : Outport
  wires:
  Mux/1 -> nu_c/1
  zero/1 -> Mux/6, Mux/5, Mux/4, Mux/3
  Product1/1 -> Mux/2
  Product/1 -> Mux/1
  V_c(m/s)/1 -> Product/2, Product1/2
  cos/1 -> Product/1
  sin/1 -> Product1/1
  beta_c(rad)/1 -> cos/1, sin/1

== system Main_Project/Hydrofoil force/deg2rad ==
  In : Inport
  Gain : Gain  Gain=k  SaturateOnIntegerOverflow=on  OutDataTypeStr=Inherit: Same as input  ParamDataTypeStr=Inherit: Same as input
  Out : Outport
  wires:
  Gain/1 -> Out/1
  In/1 -> Gain/1

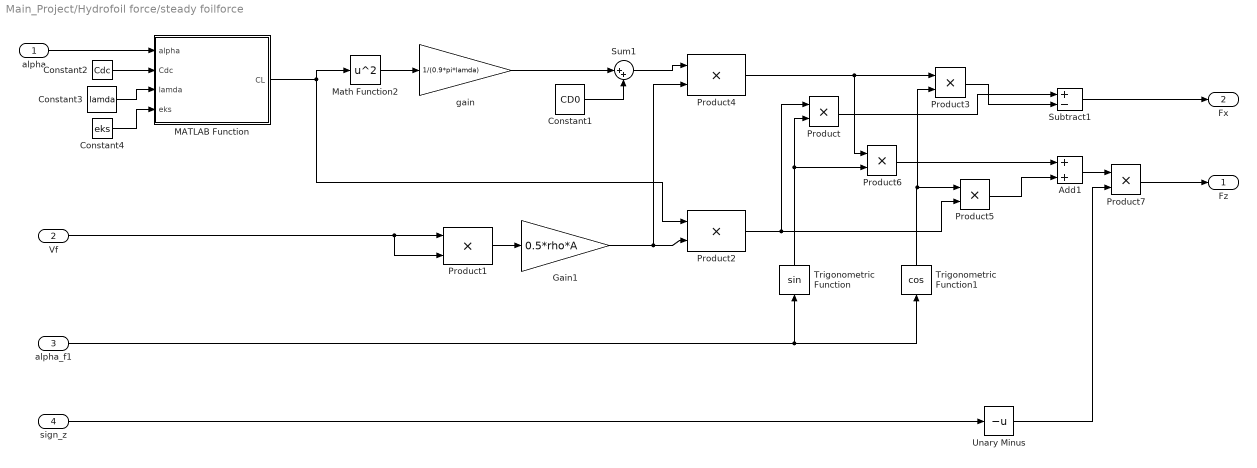
== system Main_Project/Hydrofoil force/steady foilforce ==
  alpha : Inport
  "Vf " : Inport  Port=2
  alpha_f1 : Inport  Port=3
  sign_z : Inport  Port=4
  Add1 : Sum
  Constant1 : Constant  Value=CD0
  Constant2 : Constant  Value=Cdc
  Constant3 : Constant  Value=lamda
  Constant4 : Constant  Value=eks
  Gain1 : Gain  Gain=0.5*rho*A  SaturateOnIntegerOverflow=on  OutDataTypeStr=Inherit: Same as input  ParamDataTypeStr=Inherit: Same as input
  MATLAB Function : MATLAB Function  TreatAsAtomicUnit=on
  Math Function2 : Math  Operator=square  SaturateOnIntegerOverflow=on
  Product{,3,5..7} (5 alike) : Product
  Product1 : Product  Inputs=**  SaturateOnIntegerOverflow=on  InputSameDT=on  OutDataTypeStr=Inherit: Same as first input
  Product2 : Product  SaturateOnIntegerOverflow=on  InputSameDT=on  OutDataTypeStr=Inherit: Same as first input
  Product4 : Product  SaturateOnIntegerOverflow=on  InputSameDT=on  OutDataTypeStr=Inherit: Same as first input
  Subtract1 : Sum  Inputs=+-
  Sum1 : Sum  Inputs=|++  SaturateOnIntegerOverflow=on  InputSameDT=on  OutDataTypeStr=Inherit: Same as first input
  Trigonometric Function : Trigonometry
  Trigonometric Function1 : Trigonometry  Operator=cos
  Unary Minus : UnaryMinus
  "gain " : Gain  Gain=1/(0.9*pi*lamda)  SaturateOnIntegerOverflow=on  OutDataTypeStr=Inherit: Same as input  ParamDataTypeStr=Inherit: Same as input
  Fz : Outport
  Fx : Outport  Port=2
  wires:
  Product3/1 -> Subtract1/2
  Trigonometric Function1/1 -> Product5/1, Product3/2
  alpha_f1/1 -> Trigonometric Function1/1, Trigonometric Function/1
  Trigonometric Function/1 -> Product6/2, Product/2
  Product2/1 -> Product/1, Product5/2
  Subtract1/1 -> Fx/1
  "Vf "/1 -> Product1/1, Product1/2
  Constant1/1 -> Sum1/2
  "gain "/1 -> Sum1/1
  Product/1 -> Subtract1/1
  Product1/1 -> Gain1/1
  alpha/1 -> MATLAB Function/1(alpha)
  Constant4/1 -> MATLAB Function/4(eks)
  Constant3/1 -> MATLAB Function/3(lamda)
  Constant2/1 -> MATLAB Function/2(Cdc)
  Unary Minus/1 -> Product7/2
  Product7/1 -> Fz/1
  sign_z/1 -> Unary Minus/1
  Add1/1 -> Product7/1
  Product5/1 -> Add1/2
  Product6/1 -> Add1/1
  Math Function2/1 -> "gain "/1
  Sum1/1 -> Product4/1
  Gain1/1 -> Product2/2, Product4/2
  Product4/1 -> Product3/1, Product6/1
  MATLAB Function/1(CL) -> Math Function2/1, Product2/1

== system Main_Project/Wave loads/Wave loads for heading1 ==
  eta : Inport
  psi : Inport  Port=2
  psi_wave : Inport  Port=3
  wavenum : Inport  Port=4
  Omega : Inport  Port=5
  Phase : Inport  Port=6
  Zeta_a : Inport  Port=7
  Clock : Clock
  Position phase : Subsystem  mask(Position Phase){}
      mask help: Calculate the phase delay due to the vessel LF position.
  Product1 : Product  Inputs=**  SaturateOnIntegerOverflow=on  OutDataTypeStr=Inherit: Same as first input
  Sum : Sum  Inputs=-++  SaturateOnIntegerOverflow=on
  Sum1 : Sum  Inputs=-+|
  Wave component loop : Subsystem  TreatAsAtomicUnit=on
  Width : Width  DataType=int32
  tau_WF : Outport
  tau_WD : Outport  Port=2
  wires:
  psi/1 -> Sum1/1  "psi"
  Wave component loop/2(tau_WD) -> tau_WD/1
  Sum1/1 -> Wave component loop/2(Psi_r)
  Zeta_a/1 -> Wave component loop/5(Zeta_a)
  Phase/1 -> Sum/3
  Omega/1 -> Width/1, Wave component loop/3(Omega), Product1/1
  wavenum/1 -> Position phase/2(wavenum)
  psi_wave/1 -> Sum1/2, Position phase/1(psi wave)
  eta/1 -> Position phase/3(eta LF)
  Wave component loop/1(tau_WF) -> tau_WF/1
  Product1/1 -> Sum/2
  Clock/1 -> Product1/2
  Sum/1 -> Wave component loop/4(Phase_tot)  "Phase_tot"
  Width/1 -> Wave component loop/1(number of iterations)
  Position phase/1(pos phase) -> Sum/1

== system Main_Project/Wave loads/Wave loads for heading2 ==
  eta : Inport
  psi : Inport  Port=2
  psi_wave : Inport  Port=3
  wavenum : Inport  Port=4
  Omega : Inport  Port=5
  Phase : Inport  Port=6
  Zeta_a : Inport  Port=7
  Clock : Clock
  Position phase : Subsystem  mask(Position Phase){}
      mask help: Calculate the phase delay due to the vessel LF position.
  Product1 : Product  Inputs=**  SaturateOnIntegerOverflow=on  OutDataTypeStr=Inherit: Same as first input
  Sum : Sum  Inputs=-++  SaturateOnIntegerOverflow=on
  Sum1 : Sum  Inputs=-+|
  Wave component loop : Subsystem  TreatAsAtomicUnit=on
  Width : Width  DataType=int32
  tau_WF : Outport
  tau_WD : Outport  Port=2
  wires:
  psi/1 -> Sum1/1  "psi"
  Wave component loop/2(tau_WD) -> tau_WD/1
  Sum1/1 -> Wave component loop/2(Psi_r)
  Zeta_a/1 -> Wave component loop/5(Zeta_a)
  Phase/1 -> Sum/3
  Omega/1 -> Width/1, Wave component loop/3(Omega), Product1/1
  wavenum/1 -> Position phase/2(wavenum)
  psi_wave/1 -> Sum1/2, Position phase/1(psi wave)
  eta/1 -> Position phase/3(eta LF)
  Wave component loop/1(tau_WF) -> tau_WF/1
  Product1/1 -> Sum/2
  Clock/1 -> Product1/2
  Sum/1 -> Wave component loop/4(Phase_tot)  "Phase_tot"
  Width/1 -> Wave component loop/1(number of iterations)
  Position phase/1(pos phase) -> Sum/1

== system Main_Project/Wave loads/deg to 180//180 ==
  note: x
  note: r
  x (deg) : Inport
  Constant : Constant  Value=2*180
  Gain : Gain  Gain=180  SaturateOnIntegerOverflow=on  OutDataTypeStr=Inherit: Same as input  ParamDataTypeStr=Inherit: Same as input
  Math Function : Math  Operator=rem  SaturateOnIntegerOverflow=on
  Saturation : Saturate  UpperLimit=1e10  LowerLimit=-1e10
  Sign : Signum
  Sum : Sum  Inputs=|+-  SaturateOnIntegerOverflow=on
  Sum1 : Sum  Inputs=|++  SaturateOnIntegerOverflow=on
  -180<y<180 : Outport
  wires:
  Saturation/1 -> Sum1/1, Sign/1
  x (deg)/1 -> Saturation/1
  Sign/1 -> Gain/1
  Gain/1 -> Sum/2, Sum1/2
  Sum1/1 -> Math Function/1
  Constant/1 -> Math Function/2
  Math Function/1 -> Sum/1
  Sum/1 -> -180<y<180/1

== system Main_Project/Wave loads/psi1 ==
  k : Inport
  0 or 1 : Inport  Port=2
  Gain1 : Gain  Gain=20
  Gain2 : Gain  Gain=10
  Product : Product  RndMeth=Zero
  Sum7 : Sum  Inputs=-+|
  Sum8 : Sum  Inputs=++|
  const : Constant  Value=18
  psi : Outport
  wires:
  0 or 1/1 -> Product/2
  Sum8/1 -> psi/1
  k/1 -> Gain2/1, Sum7/1
  Gain2/1 -> Sum8/1
  Product/1 -> Sum8/2
  Gain1/1 -> Product/1
  Sum7/1 -> Gain1/1
  const/1 -> Sum7/2

== system Main_Project/Wave loads/psi2 ==
  k : Inport
  0 or 1 : Inport  Port=2
  Gain1 : Gain  Gain=20
  Gain2 : Gain  Gain=10
  Product : Product  RndMeth=Zero
  Sum7 : Sum  Inputs=-+|
  Sum8 : Sum  Inputs=++|
  const : Constant  Value=18
  psi : Outport
  wires:
  0 or 1/1 -> Product/2
  Sum8/1 -> psi/1
  k/1 -> Gain2/1, Sum7/1
  Gain2/1 -> Sum8/1
  Product/1 -> Sum8/2
  Gain1/1 -> Product/1
  Sum7/1 -> Gain1/1
  const/1 -> Sum7/2

== system Main_Project/Wave loads/Wave loads for heading1/Position phase ==
  psi wave : Inport
  wavenum : Inport  Port=2
  eta LF : Inport  Port=3
  Product2 : Product  Inputs=**  SaturateOnIntegerOverflow=on  OutDataTypeStr=Inherit: Same as first input
  Product6 : Product  Inputs=**  SaturateOnIntegerOverflow=on  OutDataTypeStr=Inherit: Same as first input
  Product7 : Product  Inputs=**  SaturateOnIntegerOverflow=on  OutDataTypeStr=Inherit: Same as first input
  Sum5 : Sum  SaturateOnIntegerOverflow=on
  cos : Trigonometry  Operator=cos
  sin : Trigonometry
  x-position : Selector  IndexOptions=Index vector (dialog)  Indices=1  OutputSizes=1
  y-position : Selector  InputPortWidth=6  IndexOptions=Index vector (dialog)  Indices=2  OutputSizes=1
  pos phase : Outport
  wires:
  Sum5/1 -> Product7/1
  Product2/1 -> Sum5/1
  sin/1 -> Product2/1
  cos/1 -> Product6/1
  x-position/1 -> Product6/2
  y-position/1 -> Product2/2
  Product6/1 -> Sum5/2
  psi wave/1 -> sin/1, cos/1
  eta LF/1 -> x-position/1, y-position/1
  Product7/1 -> pos phase/1
  wavenum/1 -> Product7/2

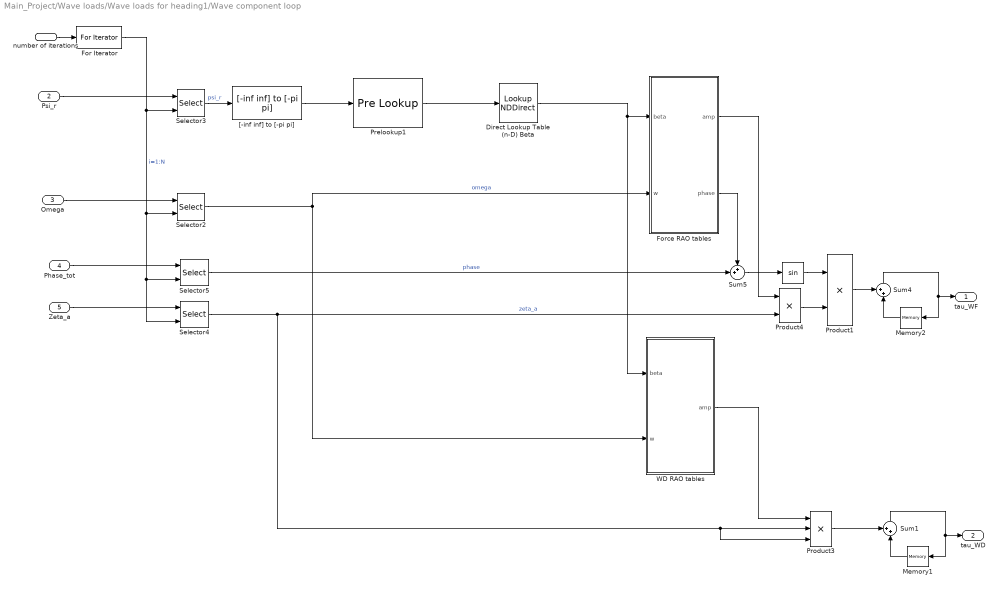
== system Main_Project/Wave loads/Wave loads for heading1/Wave component loop ==
  number of iterations : Inport
  Psi_r : Inport  Port=2
  Omega : Inport  Port=3
  Phase_tot : Inport  Port=4
  Zeta_a : Inport  Port=5
  "                " : Trigonometry
  Direct Lookup Table (n-D) Beta : LookupNDDirect  NumberOfTableDimensions=1  Table=float.headings
  For Iterator : ForIterator  ResetStates=reset  IterationSource=external  IterationVariableDataType=double
  Force RAO tables : Subsystem  mask(RAO table lookup){}
      mask help:
      | Perform 3D table lookup in 6DOF RAO amplitudes and phases, using the relative wave heading psi_r, wave frequency omega and vessel velocity vel as inputs. See documentation of the Motion RAO block or Force RAO block for details. A warning is issued if the input is outside the range spanned by the RAOs.
      |
      | Author: Oyvind N. Smogeli and Thor I. Fossen, 2005-05-03
  Memory1 : Memory  X0=[0 0 0 0 0 0]'  InheritSampleTime=on
  Memory2 : Memory  X0=[0 0 0 0 0 0]'  InheritSampleTime=on
  Prelookup1 : PreLookup  BreakpointsData=float.headings  IndexSearchMethod=Linear search  BeginIndexSearchUsingPreviousIndexResult=on  OutputOnlyTheIndex=on
  Product1 : Product  SaturateOnIntegerOverflow=on  OutDataTypeStr=Inherit: Same as first input
  Product3 : Product  Inputs=3  SaturateOnIntegerOverflow=on  OutDataTypeStr=Inherit: Same as first input
  Product4 : Product  SaturateOnIntegerOverflow=on  OutDataTypeStr=Inherit: Same as first input
  Selector{2..5} (4 alike) : Selector  IndexOptions=Index vector (port)  Indices=[1 3]  OutputSizes=1
  Sum1 : Sum  Inputs=++|  SaturateOnIntegerOverflow=on
  Sum4 : Sum  Inputs=++|  SaturateOnIntegerOverflow=on
  Sum5 : Sum  Inputs=++|  SaturateOnIntegerOverflow=on
  WD RAO tables : Subsystem  mask(RAO table lookup){}
      mask help:
      | Perform 3D table lookup in 6DOF RAO amplitudes and phases, using the relative wave heading psi_r, wave frequency omega and vessel velocity vel as inputs. See documentation of the Motion RAO block or Force RAO block for details. A warning is issued if the input is outside the range spanned by the RAOs.
      |
      | Author: Oyvind N. Smogeli and Thor I. Fossen, 2005-05-03
  "[-inf inf] to [-pi pi]" : marine_gnc/Utilities/Math Operations/[-inf inf] to [-pi pi]
  tau_WF : Outport
  tau_WD : Outport  Port=2
  wires:
  WD RAO tables/1(amp) -> Product3/1
  Force RAO tables/1(amp) -> Product4/1
  Force RAO tables/2(phase) -> Sum5/1
  Direct Lookup Table (n-D) Beta/1 -> WD RAO tables/1(beta), Force RAO tables/1(beta)
  Prelookup1/1 -> Direct Lookup Table (n-D) Beta/1
  For Iterator/1 -> Selector5/2, Selector4/2, Selector2/2, Selector3/2  "i=1:N"
  Selector2/1 -> WD RAO tables/2(w), Force RAO tables/2(w)  "omega"
  "[-inf inf] to [-pi pi]"/1 -> Prelookup1/1
  Product3/1 -> Sum1/1
  Memory1/1 -> Sum1/2
  Sum1/1 -> tau_WD/1, Memory1/1
  Product4/1 -> Product1/2
  "                "/1 -> Product1/1
  Selector3/1 -> "[-inf inf] to [-pi pi]"/1  "psi_r"
  Selector5/1 -> Sum5/2  "phase"
  Product1/1 -> Sum4/1
  Memory2/1 -> Sum4/2
  Sum4/1 -> tau_WF/1, Memory2/1
  number of iterations/1 -> For Iterator/1
  Omega/1 -> Selector2/1
  Psi_r/1 -> Selector3/1
  Phase_tot/1 -> Selector5/1
  Zeta_a/1 -> Selector4/1
  Sum5/1 -> "                "/1
  Selector4/1 -> Product3/3, Product3/2, Product4/2  "zeta_a"

== system Main_Project/Wave loads/Wave loads for heading2/Position phase ==
  psi wave : Inport
  wavenum : Inport  Port=2
  eta LF : Inport  Port=3
  Product2 : Product  Inputs=**  SaturateOnIntegerOverflow=on  OutDataTypeStr=Inherit: Same as first input
  Product6 : Product  Inputs=**  SaturateOnIntegerOverflow=on  OutDataTypeStr=Inherit: Same as first input
  Product7 : Product  Inputs=**  SaturateOnIntegerOverflow=on  OutDataTypeStr=Inherit: Same as first input
  Sum5 : Sum  SaturateOnIntegerOverflow=on
  cos : Trigonometry  Operator=cos
  sin : Trigonometry
  x-position : Selector  IndexOptions=Index vector (dialog)  Indices=1  OutputSizes=1
  y-position : Selector  InputPortWidth=6  IndexOptions=Index vector (dialog)  Indices=2  OutputSizes=1
  pos phase : Outport
  wires:
  Sum5/1 -> Product7/1
  Product2/1 -> Sum5/1
  sin/1 -> Product2/1
  cos/1 -> Product6/1
  x-position/1 -> Product6/2
  y-position/1 -> Product2/2
  Product6/1 -> Sum5/2
  psi wave/1 -> sin/1, cos/1
  eta LF/1 -> x-position/1, y-position/1
  Product7/1 -> pos phase/1
  wavenum/1 -> Product7/2

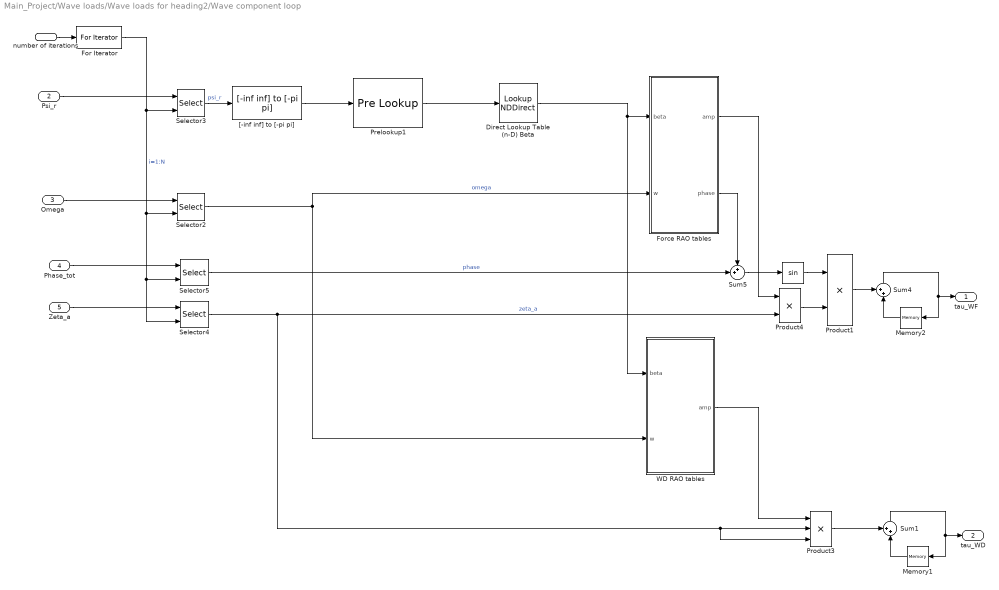
== system Main_Project/Wave loads/Wave loads for heading2/Wave component loop ==
  number of iterations : Inport
  Psi_r : Inport  Port=2
  Omega : Inport  Port=3
  Phase_tot : Inport  Port=4
  Zeta_a : Inport  Port=5
  "                " : Trigonometry
  Direct Lookup Table (n-D) Beta : LookupNDDirect  NumberOfTableDimensions=1  Table=float.headings
  For Iterator : ForIterator  ResetStates=reset  IterationSource=external  IterationVariableDataType=double
  Force RAO tables : Subsystem  mask(RAO table lookup){}
      mask help:
      | Perform 3D table lookup in 6DOF RAO amplitudes and phases, using the relative wave heading psi_r, wave frequency omega and vessel velocity vel as inputs. See documentation of the Motion RAO block or Force RAO block for details. A warning is issued if the input is outside the range spanned by the RAOs.
      |
      | Author: Oyvind N. Smogeli and Thor I. Fossen, 2005-05-03
  Memory1 : Memory  X0=[0 0 0 0 0 0]'  InheritSampleTime=on
  Memory2 : Memory  X0=[0 0 0 0 0 0]'  InheritSampleTime=on
  Prelookup1 : PreLookup  BreakpointsData=float.headings  IndexSearchMethod=Linear search  BeginIndexSearchUsingPreviousIndexResult=on  OutputOnlyTheIndex=on
  Product1 : Product  SaturateOnIntegerOverflow=on  OutDataTypeStr=Inherit: Same as first input
  Product3 : Product  Inputs=3  SaturateOnIntegerOverflow=on  OutDataTypeStr=Inherit: Same as first input
  Product4 : Product  SaturateOnIntegerOverflow=on  OutDataTypeStr=Inherit: Same as first input
  Selector{2..5} (4 alike) : Selector  IndexOptions=Index vector (port)  Indices=[1 3]  OutputSizes=1
  Sum1 : Sum  Inputs=++|  SaturateOnIntegerOverflow=on
  Sum4 : Sum  Inputs=++|  SaturateOnIntegerOverflow=on
  Sum5 : Sum  Inputs=++|  SaturateOnIntegerOverflow=on
  WD RAO tables : Subsystem  mask(RAO table lookup){}
      mask help:
      | Perform 3D table lookup in 6DOF RAO amplitudes and phases, using the relative wave heading psi_r, wave frequency omega and vessel velocity vel as inputs. See documentation of the Motion RAO block or Force RAO block for details. A warning is issued if the input is outside the range spanned by the RAOs.
      |
      | Author: Oyvind N. Smogeli and Thor I. Fossen, 2005-05-03
  "[-inf inf] to [-pi pi]" : marine_gnc/Utilities/Math Operations/[-inf inf] to [-pi pi]
  tau_WF : Outport
  tau_WD : Outport  Port=2
  wires:
  WD RAO tables/1(amp) -> Product3/1
  Force RAO tables/1(amp) -> Product4/1
  Force RAO tables/2(phase) -> Sum5/1
  Direct Lookup Table (n-D) Beta/1 -> WD RAO tables/1(beta), Force RAO tables/1(beta)
  Prelookup1/1 -> Direct Lookup Table (n-D) Beta/1
  For Iterator/1 -> Selector5/2, Selector4/2, Selector2/2, Selector3/2  "i=1:N"
  Selector2/1 -> WD RAO tables/2(w), Force RAO tables/2(w)  "omega"
  "[-inf inf] to [-pi pi]"/1 -> Prelookup1/1
  Product3/1 -> Sum1/1
  Memory1/1 -> Sum1/2
  Sum1/1 -> tau_WD/1, Memory1/1
  Product4/1 -> Product1/2
  "                "/1 -> Product1/1
  Selector3/1 -> "[-inf inf] to [-pi pi]"/1  "psi_r"
  Selector5/1 -> Sum5/2  "phase"
  Product1/1 -> Sum4/1
  Memory2/1 -> Sum4/2
  Sum4/1 -> tau_WF/1, Memory2/1
  number of iterations/1 -> For Iterator/1
  Omega/1 -> Selector2/1
  Psi_r/1 -> Selector3/1
  Phase_tot/1 -> Selector5/1
  Zeta_a/1 -> Selector4/1
  Sum5/1 -> "                "/1
  Selector4/1 -> Product3/3, Product3/2, Product4/2  "zeta_a"
